simulink library "DelayAndTargetOverlaying"  (R2018a)
settings: Solver=VariableStepAuto  StartTime=0.0  StopTime=10.0  RelTol=1e-3
undefined symbols (not defined in the file): fF, xs, ys
libraries: visiontextngfix x1
settings Model: Creator=Sky  LastModifiedBy=Sky

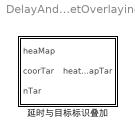
== system DelayAndTargetOverlaying ==
  延时与目标标识叠加 : Subsystem  mask{lW=1, xs=xs, ys=ys, tDelay=0.5, fF=fF}
      mask prompts: lW "window length"
      mask help:
      | 为输入的雷达成像图叠加目标标识，这里用一个宽度为window length的正方形指示目标位置。
      |
      | 端口说明：
      | heatMap：从“雷达成像和定位”模块输出的雷达成像。行对应y方向，列对应x方向。
      | coorTar：n行2列的矩阵，n个目标的坐标，单位（m）。第1列为x坐标，第2列为y坐标。前nTar个坐标为有效坐标。
      | nTar：目标的个数。
      | heatMapTar：叠加了目标标识的雷达图像。
      |
      | 参数说明：
      | window length：正方形标识的宽度
      | xs：x坐标序列，单位（m）。对应heatMap的列。
      | ys：y坐标序列，单位（m）。对应heatMap的行。
      | tDelay：如果coorTar端口输入的目标坐标经过“坐标异常值剔除和滤波”模块的处理，会对目标坐标引入一定延时。此参数用于设置对heatMap的延时，以保证目标标识无偏移地叠加到heatMap上。
      | fF：帧率。
      mask TypeOptions lW: 目标标识叠加/lW
      mask TypeOptions xs: 目标标识叠加/xs
      mask TypeOptions ys: 目标标识叠加/ys

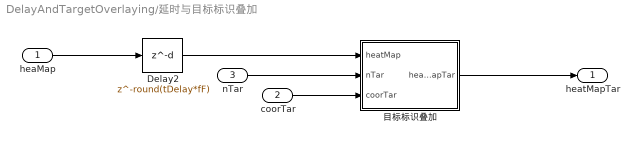
== system DelayAndTargetOverlaying/延时与目标标识叠加 ==
  heaMap : Inport
  coorTar : Inport  Port=2
  nTar : Inport  Port=3
  Delay2 : Delay  DelayLength=round(tDelay*fF)  InitialCondition=0
  目标标识叠加 : Subsystem  mask{lW=lW, xs=xs, ys=ys}
      mask prompts: lW "window length"
  heatMapTar : Outport
  wires:
  目标标识叠加/1(heatMapTar) -> heatMapTar/1
  heaMap/1 -> Delay2/1
  Delay2/1 -> 目标标识叠加/1(heatMap)
  nTar/1 -> 目标标识叠加/2(nTar)
  coorTar/1 -> 目标标识叠加/3(coorTar)

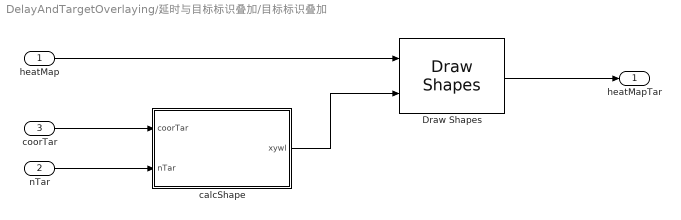
== system DelayAndTargetOverlaying/延时与目标标识叠加/目标标识叠加 ==
  heatMap : Inport
  nTar : Inport  Port=2
  coorTar : Inport  Port=3
  Draw Shapes : visiontextngfix/Draw Shapes  shape=Rectangles  fill=off  lineWidth=1  fillClrSource=Specify via dialog  display=White  intensity=200  color=[200 255 100]  opacity=0.6  viewport=Entire image  antialiasing=off  inType=Obsolete  imagePorts=One multidimensional signal  prodOutputMode=Binary point scaling  prodOutputWordLength=32  prodOutputFracLength=14  memoryMode=Specify word length  memoryWordLength=16  memoryFracLength=15  roundingMode=Floor  overflowMode=off
      settings: SourceProductName=Computer Vision System Toolbox
  calcShape : MATLAB Function  TreatAsAtomicUnit=on
  heatMapTar : Outport
  wires:
  calcShape/1(xywl) -> Draw Shapes/2
  Draw Shapes/1 -> heatMapTar/1
  nTar/1 -> calcShape/2(nTar)
  heatMap/1 -> Draw Shapes/1
  coorTar/1 -> calcShape/1(coorTar)

== matlab function DelayAndTargetOverlaying/延时与目标标识叠加/目标标识叠加/calcShape ==
  data: coorTar input; xs parameter; ys parameter; xywl output size=[size(coorTar,1),4]; lW parameter; nTar input
function xywl = calcShape(coorTar, xs, ys, lW, nTar)
if nTar~=0
    iXTar=interp1(xs,1:length(xs),coorTar(1:nTar,1),'nearest');
    iYTar=interp1(ys,1:length(ys),coorTar(1:nTar,2),'nearest');
    lXW=lW/diff(xs(1:2));
    lYW=lW/diff(ys(1:2));
    xywl=[iXTar-lXW/2 iYTar-lYW/2 repmat([lXW lYW],nTar,1)];
else
    xywl=zeros(0,4,'single');
end
